simulink model "spwm25hz"  (Simulink 7.4)
settings: Solver=ode15s  StartTime=0.0  StopTime=.04  MaxStep=0.000001  MinStep=0.00000001  RelTol=1e-5
libraries: powerlib x22, simulink x1
settings Model: Creator=Administrator  LastModifiedBy=dell
settings SolverCC: InitialStep=0.00000001
settings OptimizationCC: InitFltsAndDblsToZero=on
settings DebuggingCC: SaveWithParameterizedLinksMsg=none  SignalResolutionControl=TryResolveAllWithWarning
settings GRTTargetCC: TargetFcnLib=ansi_tfl_tmw.mat

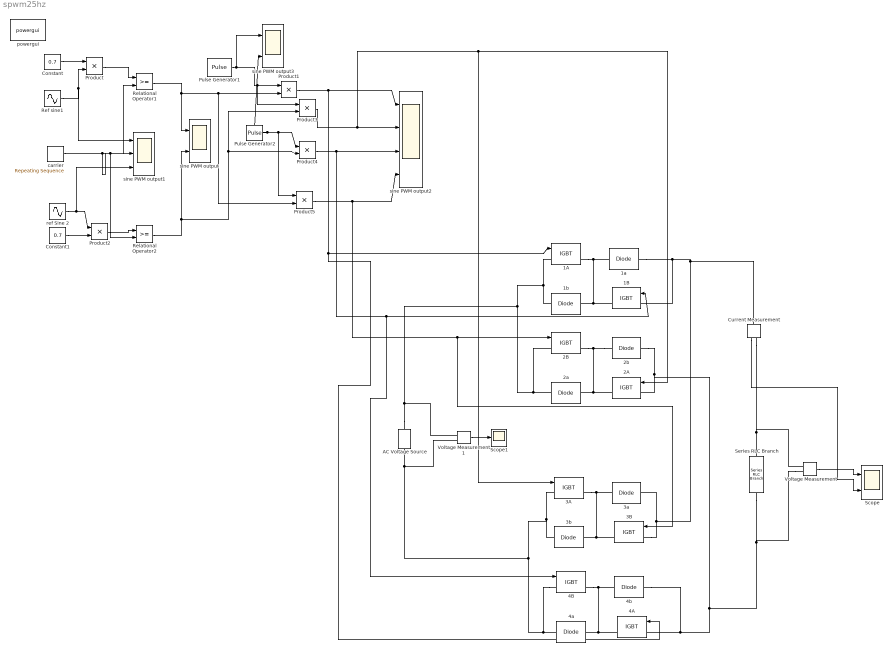
== system spwm25hz ==
  1A : powerlib/Power Electronics/IGBT  DialogController=POWERSYS.PowerSysDialog  SystemSampleTime=-1  Ron=0.001  Lon=0  Vf=1  Tf=1e-6  Tt=2e-6  IC=0  Rs=1e5  Cs=inf  Measurements=on
  1B : powerlib/Power Electronics/IGBT  DialogController=POWERSYS.PowerSysDialog  SystemSampleTime=-1  Ron=0.001  Lon=0  Vf=1  Tf=1e-6  Tt=2e-6  IC=0  Rs=1e5  Cs=inf  Measurements=on
  1a : powerlib/Power Electronics/Diode  DialogController=POWERSYS.PowerSysDialog  SystemSampleTime=-1  Ron=0.001  Lon=0  Vf=0.8  IC=0  UseSnubber=off  Rs=500  Cs=250e-9  Measurements=off
  1b : powerlib/Power Electronics/Diode  DialogController=POWERSYS.PowerSysDialog  SystemSampleTime=-1  Ron=0.001  Lon=0  Vf=0.8  IC=0  UseSnubber=off  Rs=500  Cs=250e-9  Measurements=off
  2A : powerlib/Power Electronics/IGBT  DialogController=POWERSYS.PowerSysDialog  SystemSampleTime=-1  Ron=0.001  Lon=0  Vf=1  Tf=1e-6  Tt=2e-6  IC=0  Rs=1e5  Cs=inf  Measurements=on
  2B : powerlib/Power Electronics/IGBT  DialogController=POWERSYS.PowerSysDialog  SystemSampleTime=-1  Ron=0.001  Lon=0  Vf=1  Tf=1e-6  Tt=2e-6  IC=0  Rs=1e5  Cs=inf  Measurements=on
  2a : powerlib/Power Electronics/Diode  DialogController=POWERSYS.PowerSysDialog  SystemSampleTime=-1  Ron=0.001  Lon=0  Vf=0.8  IC=0  UseSnubber=off  Rs=500  Cs=250e-9  Measurements=off
  2b : powerlib/Power Electronics/Diode  DialogController=POWERSYS.PowerSysDialog  SystemSampleTime=-1  Ron=0.001  Lon=0  Vf=0.8  IC=0  UseSnubber=off  Rs=500  Cs=250e-9  Measurements=off
  3A : powerlib/Power Electronics/IGBT  DialogController=POWERSYS.PowerSysDialog  SystemSampleTime=-1  Ron=0.001  Lon=0  Vf=1  Tf=1e-6  Tt=2e-6  IC=0  Rs=1e5  Cs=inf  Measurements=on
  3B : powerlib/Power Electronics/IGBT  DialogController=POWERSYS.PowerSysDialog  SystemSampleTime=-1  Ron=0.001  Lon=0  Vf=1  Tf=1e-6  Tt=2e-6  IC=0  Rs=1e5  Cs=inf  Measurements=on
  3a : powerlib/Power Electronics/Diode  DialogController=POWERSYS.PowerSysDialog  SystemSampleTime=-1  Ron=0.001  Lon=0  Vf=0.8  IC=0  UseSnubber=off  Rs=500  Cs=250e-9  Measurements=off
  3b : powerlib/Power Electronics/Diode  DialogController=POWERSYS.PowerSysDialog  SystemSampleTime=-1  Ron=0.001  Lon=0  Vf=0.8  IC=0  UseSnubber=off  Rs=500  Cs=250e-9  Measurements=off
  4A : powerlib/Power Electronics/IGBT  DialogController=POWERSYS.PowerSysDialog  SystemSampleTime=-1  Ron=0.001  Lon=0  Vf=1  Tf=1e-6  Tt=2e-6  IC=0  Rs=1e5  Cs=inf  Measurements=on
  4B : powerlib/Power Electronics/IGBT  DialogController=POWERSYS.PowerSysDialog  SystemSampleTime=-1  Ron=0.001  Lon=0  Vf=1  Tf=1e-6  Tt=2e-6  IC=0  Rs=1e5  Cs=inf  Measurements=on
  4a : powerlib/Power Electronics/Diode  DialogController=POWERSYS.PowerSysDialog  SystemSampleTime=-1  Ron=0.001  Lon=0  Vf=0.8  IC=0  UseSnubber=off  Rs=500  Cs=250e-9  Measurements=off
  4b : powerlib/Power Electronics/Diode  DialogController=POWERSYS.PowerSysDialog  SystemSampleTime=-1  Ron=0.001  Lon=0  Vf=0.8  IC=0  UseSnubber=off  Rs=500  Cs=250e-9  Measurements=off
  AC Voltage Source : powerlib/Electrical Sources/AC Voltage Source  DialogController=POWERSYS.PowerSysDialog  SystemSampleTime=-1  Amplitude=50  Phase=0  Frequency=50  SampleTime=0  Measurements=None
  Constant : Constant  Value=0.7  OutDataType=sfix(16)  OutScaling=2^0
  Constant1 : Constant  Value=0.7  OutDataType=sfix(16)  OutScaling=2^0
  Current Measurement : powerlib/Measurements/Current Measurement  DialogController=POWERSYS.PowerSysDialog  SystemSampleTime=-1  PhasorSimulation=off  OutputType=Complex  PSBequivalent=0
  Product{,1..5} (6 alike) : Product  OutDataType=sfix(16)  OutScaling=2^0  RndMeth=Zero
  Pulse Generator1 : DiscretePulseGenerator  PulseType=Time based  Amplitude=1  Period=.04  PulseWidth=50  PhaseDelay=0  SampleTime=1
  Pulse Generator2 : DiscretePulseGenerator  PulseType=Time based  Amplitude=1  Period=.04  PulseWidth=50  PhaseDelay=0.02  SampleTime=1
  Ref sine1 : Sin  Amplitude=50  Bias=0  Frequency=100*pi  Phase=0  Samples=10  SampleTime=0  Offset=0
  Relational Operator1 : RelationalOperator  LogicOutDataTypeMode=boolean  OutDataTypeStr=boolean
  Relational Operator2 : RelationalOperator  LogicOutDataTypeMode=boolean  OutDataTypeStr=boolean
  Scope : Scope  NumInputPorts=2
      settings: TimeRange=0.5  YMin=-250~-22.5  YMax=250~22.5  SaveName=ScopeData5
  Scope1 : Scope
  Series RLC Branch : powerlib/Elements/Series RLC Branch  DialogController=POWERSYS.PowerSysDialog  PhysicalDomain=powersysdomain  SubClassName=unknown  LeftPortType=p1  RightPortType=p1  LConnTagsString=__new0  RConnTagsString=__new0  BranchType=R  Resistance=10  Inductance=1e-3  SetiL0=off  InitialCurrent=0  Capacitance=1e-6  Setx0=off  InitialVoltage=0  Measurements=None
  Voltage Measurement : powerlib/Measurements/Voltage Measurement  DialogController=POWERSYS.PowerSysDialog  SystemSampleTime=-1  PhasorSimulation=off  OutputType=Complex  PSBequivalent=0
  Voltage Measurement1 : powerlib/Measurements/Voltage Measurement  DialogController=POWERSYS.PowerSysDialog  SystemSampleTime=-1  PhasorSimulation=off  OutputType=Complex  PSBequivalent=0
  "carrier " : simulink/Sources/Repeating Sequence  SystemSampleTime=-1  rep_seq_t=[0 0.0001 0.0002]  rep_seq_y=[0 40 0]
  powergui : powerlib/powergui  Priority=1  SystemSampleTime=-1  SimulationMode=Continuous  SampleTime=50e-6  frequency=60  SPID=off  DisableSnubberDevices=off  DisableRonSwitches=off  DisableVfSwitches=off  SwTol=0  Interpol=off  frequencyindice=50  echomessages=off  HookPort=off  DisplayEquations=off  FunctionMessages=off  EnableUseOfTLC=off  x0status=blocks  RestoreLinks=warning  Frange=[0:2:500]  Ylog=off  Xlog=on  ShowGrid=off  save=off  variable=ZData  ZoomFFT=off  StartTime=0.0  cycles=1  DisplayStyle=1  fundamental=60  FreqAxis=off  MaxFrequency=1000  frequencyindicesteady=1  RmsSteady=1  display=off  Ts=0  methode=off
  ref Sine 2 : Sin  Amplitude=50  Bias=0  Frequency=100*pi  Phase=pi  Samples=10  SampleTime=0  Offset=0
  sine PWM output : Scope  NumInputPorts=2
      settings: Tag=sine PWM output  YMin=0~0  YMax=2~2  MaxDataPoints=500000
  sine PWM output1 : Scope  NumInputPorts=3
      settings: Tag=sine PWM output  YMin=0~0~-5  YMax=2~2~5  SaveName=ScopeData2  MaxDataPoints=500000
  sine PWM output2 : Scope  NumInputPorts=4
      settings: Tag=sine PWM output  YMin=-2~-2~-2~-2  YMax=2~2~2~2  SaveName=ScopeData3  MaxDataPoints=500000
  sine PWM output3 : Scope  NumInputPorts=2
      settings: Tag=sine PWM output  YMin=-2~-3  YMax=2~3  SaveName=ScopeData4  MaxDataPoints=500000
  wires:
  Ref sine1/1 -> Product/2, sine PWM output1/1
  "carrier "/1 -> Relational Operator2/2, Relational Operator1/2, sine PWM output1/2
  ref Sine 2/1 -> Product2/1, sine PWM output1/3
  Product2/1 -> Relational Operator2/1
  Product/1 -> Relational Operator1/1
  Constant1/1 -> Product2/2
  Constant/1 -> Product/1
  Relational Operator1/1 -> sine PWM output/1, Product1/2, Product5/2
  Relational Operator2/1 -> sine PWM output/2, Product3/2, Product4/2
  Pulse Generator1/1 -> sine PWM output3/1, Product1/1, Product3/1
  Pulse Generator2/1 -> sine PWM output3/2, Product5/1, Product4/1
  Product1/1 -> sine PWM output2/1, 1A/1, 4A/1
  Product5/1 -> sine PWM output2/4, 2B/1, 3B/1
  Product3/1 -> sine PWM output2/2, 2A/1, 3A/1
  Product4/1 -> sine PWM output2/3, 1B/1, 4B/1
  Voltage Measurement/1 -> Scope/1
  Voltage Measurement1/1 -> Scope1/1
  Current Measurement/1 -> Scope/2
  connections:
  2b/LConn1 -- 2a/LConn1 -- 2A/RConn1 -- 2B/RConn1
  1b/LConn1 -- 1B/RConn1 -- 1A/RConn1 -- 1a/LConn1
  AC Voltage Source/RConn1 -- 1b/RConn1 -- 1A/LConn1 -- 2a/RConn1 -- 2B/LConn1 -- Voltage Measurement1/LConn1
  3b/LConn1 -- 3B/RConn1 -- 3A/RConn1 -- 3a/LConn1
  4B/LConn1 -- 4a/RConn1 -- AC Voltage Source/LConn1 -- Voltage Measurement1/LConn2 -- 3b/RConn1 -- 3A/LConn1
  3a/RConn1 -- 1a/RConn1 -- 1B/LConn1 -- Current Measurement/LConn1 -- 3B/LConn1
  4a/LConn1 -- 4A/RConn1 -- 4B/RConn1 -- 4b/LConn1
  Voltage Measurement/LConn2 -- Series RLC Branch/RConn1 -- 2b/RConn1 -- 2A/LConn1 -- 4A/LConn1 -- 4b/RConn1
  Current Measurement/RConn1 -- Voltage Measurement/LConn1 -- Series RLC Branch/LConn1
